simulink model "Synchronousfor2016a"  (R2016a)
settings: Solver=VariableStepAuto  SolverMode=SingleTasking  StartTime=0.0  StopTime=1  MaxStep=1e-4  RelTol=1e-3
undefined symbols (not defined in the file or in its folder): powergui
libraries: powerlib x3, simulink x1
settings Model: Creator=80573  LastModifiedBy=B210b
settings DebuggingCC: SFUnexpectedBacktrackingDiag=error  SFNoUnconditionalDefaultTransitionDiag=error
settings GRTTargetCC: TargetLangStandard=C99 (ISO)  GeneratePreprocessorConditionals=Use local settings
settings ConfigComp: CovMetricSettings=dwe  CovHtmlReporting=off  CovSaveCumulativeToWorkspaceVar=off  CovSaveSingleToWorkspaceVar=off  CovExternalEMLEnable=on

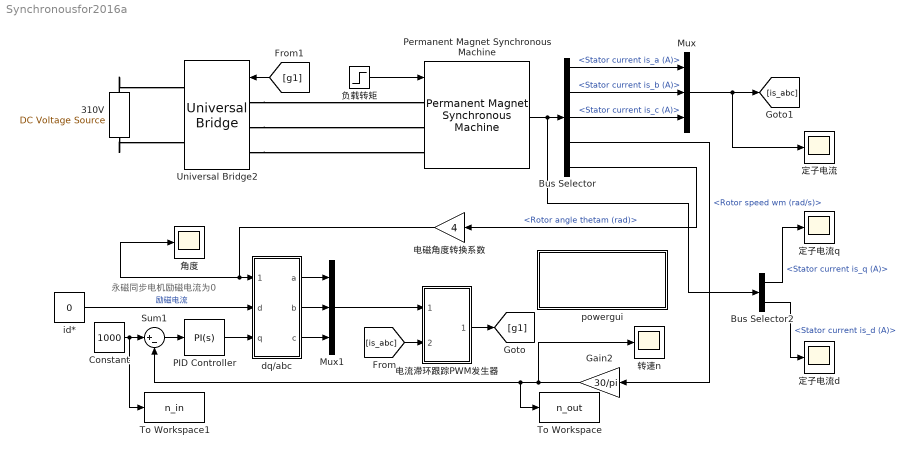
== system Synchronousfor2016a ==
  note: 永磁同步电机励磁电流为0
  310V : powerlib/Electrical Sources/DC Voltage Source  Amplitude=310  Measurements=None
  Bus Selector : BusSelector  OutputSignals=Stator current is_a (A),Stator current is_b (A),Stator current is_c (A),Rotor speed wm (rad/s),Rotor angle thetam (rad)
  Bus Selector2 : BusSelector  OutputSignals=Stator current is_q (A),Stator current is_d (A)
  Constant : Constant  Value=1000
  Gain2 : Gain  Gain=30/pi
  Mux : Mux  Inputs=3
  Mux1 : Mux  Inputs=3
  PID Controller : simulink/Continuous/PID Controller  Controller=PI  Form=Parallel  TimeDomain=Continuous-time  SampleTime=-1  IntegratorMethod=Forward Euler  FilterMethod=Forward Euler  ControllerParametersSource=internal  P=0.05  I=8  D=0  UseFilter=on  N=100  InitialConditionSource=internal  InitialConditionForIntegrator=0  InitialConditionForFilter=0  DifferentiatorICPrevScaledInput=0  ExternalReset=none  TrackingMode=off  Kt=1  LimitOutput=off  UpperSaturationLimit=200  LowerSaturationLimit=-inf  LinearizeAsGain=on  AntiWindupMode=none  Kb=1  POutMin=[]  POutMax=[]  IOutMin=[]  IOutMax=[]  DOutMin=[]  DOutMax=[]  NOutMin=[]  NOutMax=[]  SumOutMin=[]  SumOutMax=[]  SaturationOutMin=[]  SaturationOutMax=[]  PParamMin=[]  PParamMax=[]  IParamMin=[]  IParamMax=[]  DParamMin=[]  DParamMax=[]  NParamMin=[]  NParamMax=[]  KbParamMin=[]  KbParamMax=[]  KtParamMin=[]  KtParamMax=[]  KbOutMin=[]  KbOutMax=[]  KtOutMin=[]  KtOutMax=[]  IntegratorOutMin=[]  IntegratorOutMax=[]  FilterOutMin=[]  FilterOutMax=[]  SumI1OutMin=[]  SumI1OutMax=[]  SumI2OutMin=[]  SumI2OutMax=[]  SumI3OutMin=[]  SumI3OutMax=[]  SumDOutMin=[]  SumDOutMax=[]  DifferentiatorOutMin=[]  DifferentiatorOutMax=[]  IntegratorContinuousStateAttributes=''  IntegratorStateMustResolveToSignalObject=off  IntegratorRTWStateStorageClass=Auto  FilterContinuousStateAttributes=''  FilterStateMustResolveToSignalObject=off  FilterRTWStateStorageClass=Auto
  Permanent Magnet Synchronous Machine : powerlib/Machines/Permanent Magnet Synchronous Machine  NbPhases=3  FluxDistribution=Sinusoidal  RotorType=Salient-pole  MechanicalLoad=Torque Tm  PresetModel=No  ShowDetailedParameters=on  MeasurementBus=off  Resistance=2.785  Inductance=8.5e-3  dqInductances=[0.0085 0.0085]  La=0.02682  MachineConstant=Flux linkage established by magnets (V.s)  Flux=0.175  VoltageCst=126.966  TorqueCst=1.05  Flat=120  Mechanical=[0.001 0.008 4 0]  PolePairs=2  InitialConditions=[0,0, 0,0]  InitialConditions5ph=[0 0 0 0 0 0]  RefAngle=Aligned with phase A axis (original Park)  IterativeDiscreteModel=Trapezoidal non iterative  TsBlock=-1  TsPowergui=0
  Sum1 : Sum  Inputs=|+-
  To Workspace : ToWorkspace  VariableName=n_out  SampleTime=-1
  To Workspace1 : ToWorkspace  VariableName=n_in  SampleTime=-1
  Universal Bridge2 : powerlib/Power Electronics/Universal Bridge  Arms=3  SnubberResistance=1e5  SnubberCapacitance=inf  Device=IGBT / Diodes  Ron=1e-3  Lon=0  ForwardVoltages="[  0  0  ]"  ForwardVoltage=0  GTOparameters=[ 10e-6 , 20e-6 ]  IGBTparameters=[ 1e-6 , 2e-6 ]  Measurements=None  Measurements_2=None  converterType=Rectifier
  dq/abc : Subsystem
  id* : Constant  Value=0
  powergui : Subsystem  AncestorBlock=powerlib/powergui  DialogController=POWERSYS.PowerSysDialog  InitFcn=powergui( 'InitFcn_Callback' , gcb , 0 , [ ] );  mask(PSB option menu block){SimulationMode=Continuous, SampleTime=0.00001, frequency=50, Iterations=50, frequencyindice=0, Pbase=100e6, ErrMax=1e-4, UnitsV=kV, UnitsW=MW, buscounter=0, FunctionMessages=off, echomessages=off, EnableUseOfTLC=off, CurrentSourceSwitches=off, DisableSnubberDevices=off, DisableRonSwitches=off, DisableVfSwitches=off, DisplayEquations=off, AutomaticDiscreteSolvers=off, SolverType=Tustin/Backward Euler (TBE), Interpol=off, ExternalGateDelay=off, methode=off, Ts=100, x0status=zero, SPID=on, SwTol=0, HookPort=off, NonlinearTolerance=1e-4, nMaxIteration=100, ContinueOnMaxIteration=off, RestoreLinks=warning, ResistiveCurrentMeasurement=off, Frange=[0:2:500], Ylog=off, Xlog=on, ShowGrid=off, save=off, variable=ZData, structure=0, ZoomFFT=on, StartTime=0.0, cycles=1, DisplayStyle=1, fundamental=60, FreqAxis=off, MaxFrequency=1000, frequencyindicesteady=1, RmsSteady=1, display=off}
      mask prompts: SimulationMode "Simulation type:"; SampleTime "Sample time (s):"; frequency "Frequency (Hz):"; Iterations "Max iterations"; frequencyindice "Frequency (Hz)"; Pbase "Base power (VA)"; ErrMax "PQ tolerance (pu)"; UnitsV "Voltage units"; UnitsW "Power units"; buscounter "Load flow bus counter"; FunctionMessages "Disable Specialized Power Systems warnings"; echomessages "Display Specialized Power Systems compilation messages"; EnableUseOfTLC "Use TLC file when in Accelerator Simulation Mode and for code generation"; CurrentSourceSwitches "Disable ideal switching"; DisableSnubberDevices "Disable snubbers in switching devices"; DisableRonSwitches "Disable Ron resistances in switching devices"; DisableVfSwitches "Disable forward voltages in switching devices"; DisplayEquations "Display circuit differential equations"; AutomaticDiscreteSolvers "Automatically handle Discrete solver and Advanced tab solver settings of blocks"; SolverType "Discrete solver"; Interpol "Interpolate switching events"; ExternalGateDelay "Use time-stamped gate signals"; methode "Store switching topologies"; Ts "Buffer size (MBytes):"; x0status "Start simulation with initial electrical states from:"; SPID "Use ideal switching devices"; SwTol "Switch tolerance"; HookPort "Allow multiple powergui blocks"; NonlinearTolerance "Solver tolerance"; nMaxIteration "Maximum number of iterations"; ContinueOnMaxIteration "Continue Simulation if maximum number of iterations is reached"; RestoreLinks "Restore disabled links of Simscape Power Systems ST blocks:"; ResistiveCurrentMeasurement "Use non ideal current measurement blocks (1e-4Ohm internal resistance)"; Frange "Frequency Range"; Ylog "Log impedance"; Xlog "log Frequency"; ShowGrid "grid"; save "Save Data To Workspace"; variable "Variable Name"; structure "Structure Name (PSBFFTSCOPE)"; ZoomFFT "ZoomFFT (PSBFFTSCOPE)"; StartTime "Start Time (PSBFFTSCOPE)"; cycles "Cycles (PSBFFTSCOPE)"; DisplayStyle "Display style (PSBFFTSCOPE)"; fundamental "Fundamental (PSBFFTSCOPE)"; FreqAxis "Frequency Axis (PSBFFTSCOPE)"; MaxFrequency "Max Frequency (PSBFFTSCOPE)"; frequencyindicesteady "Frequency indice (STEADYSTATE)"; RmsSteady "RMS display (STEADYSTATE)"; display "Display Results"
      mask help: Set simulation type, simulation parameters, and preferences.
      mask init:
      | dispMessage = powergui('MaskInitialization',gcb,SimulationMode,SampleTime);
      settings: PreSaveFcn=powergui( 'PreSaveFcn_Callback' , gcb , [ ] , [ ] );  OpenFcn=sps_rtmsupport('OpenFcn',gcbh)
      mask Help: helpview(psbhelp)
      mask TypeOptions SimulationMode: Continuous | Discrete | Phasor
      mask Callback SimulationMode: powergui('SimulationType',[],[],gcb);
      mask TypeOptions UnitsV: V | kV
      mask TypeOptions UnitsW: W | kW | MW
      mask Callback CurrentSourceSwitches: powergui('SimulationType',[],[],gcb);
      mask Callback AutomaticDiscreteSolvers: powergui('SimulationType',[],[],gcb);
      mask TypeOptions SolverType: Tustin/Backward Euler (TBE) | Tustin | Backward Euler
      mask Callback SolverType: powergui('SimulationType',[],[],gcb);
      mask Callback Interpol: powergui('SimulationType',[],[],gcb);
      mask Callback ExternalGateDelay: powergui('SimulationType',[],[],gcb);
      mask Callback methode: powergui('SimulationType',[],[],gcb);
      mask TypeOptions x0status: blocks | steady | zero
      mask TypeOptions RestoreLinks: yes | warning | no
      mask Callback display: sps_rtmsupport('parametereditingmodes',gcbh) % Will be executed last in parameter callbacks to ensure mask enable consistency
      mask DialogControl AutoSolverNote Prompt: The Simulation type parameter is governed by Simulink. To access the Powergui solver settings, unselect auto (Automatic solver selection) solver in the Simulink solver options.
      mask DialogControl SteadyState Prompt: Steady-State
      mask DialogControl SteadyState Callback:
      | close_system(gcb)
      | power_steadystate(bdroot(gcb),gcb);
      mask DialogControl InitialState Prompt: Initial State
      mask DialogControl InitialState Callback:
      | close_system(gcb)
      | power_initstates(bdroot(gcb),gcb)
      mask DialogControl MachineInitialization Prompt: Machine Initialization
      mask DialogControl MachineInitialization Callback:
      | close_system(gcb)
      | power_loadflow(bdroot(gcb),gcb)
      mask DialogControl ImpedanceMeasurement Prompt: Impedance Measurement
      mask DialogControl ImpedanceMeasurement Callback:
      | close_system(gcb)
      | power_zmeter(bdroot(gcb),gcb)
      mask DialogControl FFTAnalysis Prompt: FFT Analysis
      mask DialogControl FFTAnalysis Callback:
      | close_system(gcb)
      | power_fftscope(bdroot(gcb),gcb)
      mask DialogControl LinearSystemAnalyzer Prompt: Use Linear System Analyzer
      mask DialogControl LinearSystemAnalyzer Callback:
      | close_system(gcb)
      | power_ltiview(bdroot(gcb),gcb)
      mask DialogControl HysteresisDesign Prompt: Hysteresis Design
      mask DialogControl HysteresisDesign Callback:
      | close_system(gcb)
      | power_hysteresis(bdroot(gcb),gcb)
      mask DialogControl RLCLineParameters Prompt: RLC Line Parameters
      mask DialogControl RLCLineParameters Callback:
      | close_system(gcb)
      | power_lineparam(bdroot(gcb),gcb)
      mask DialogControl GenerateReprot Prompt: Generate Report
      mask DialogControl GenerateReprot Callback:
      | close_system(gcb)
      | power_report(bdroot(gcb),gcb)
      mask DialogControl Control14 Prompt: Customize SPS blocks
      mask DialogControl Control14 Callback:
      | close_system(gcb);
      | power_customize;
      mask DialogControl LoadFlow Prompt: Load Flow
      mask DialogControl LoadFlow Callback:
      | close_system(gcb)
      | power_loadflow('-v2',bdroot(gcb))
      mask DialogControl Container14 Prompt: Load flow settings
      mask DialogControl Solver Prompt: Solver
      mask DialogControl SolverDetails Prompt: Solver details for nonlinear elements
      mask Display: color('blue'),disp(dispMessage)
  定子电流 : Scope
  定子电流d : Scope
  定子电流q : Scope
  电流滞环跟踪PWM发生器 : Subsystem
  电磁角度转换系数 : Gain  Gain=4
  角度 : Scope
  负载转矩 : Step  Time=0.02  Before=4  After=10  SampleTime=0
  转速n : Scope
  wires:
  负载转矩/1 -> Permanent Magnet Synchronous Machine/1
  Permanent Magnet Synchronous Machine/1 -> Bus Selector2/1, Bus Selector/1
  Bus Selector/1 -> Mux/1  "<Stator current is_a (A)>"
  Bus Selector/2 -> Mux/2  "<Stator current is_b (A)>"
  Bus Selector/3 -> Mux/3  "<Stator current is_c (A)>"
  Bus Selector/4 -> Gain2/1  "<Rotor speed wm (rad/s)>"
  Bus Selector/5 -> 电磁角度转换系数/1  "<Rotor angle thetam (rad)>"
  Constant/1 -> To Workspace1/1, Sum1/1
  id*/1 -> dq/abc/2(d)  "励磁电流"
  Mux/1 -> 定子电流/1, [is_abc]
  电流滞环跟踪PWM发生器/1(pulse) -> [g1]
  dq/abc/1(a) -> Mux1/1
  dq/abc/2(b) -> Mux1/2
  dq/abc/3(c) -> Mux1/3
  Mux1/1 -> 电流滞环跟踪PWM发生器/1(Iabc*)
  [is_abc] -> 电流滞环跟踪PWM发生器/2(Iabc)
  电磁角度转换系数/1 -> 角度/1, dq/abc/1(theta)
  [g1] -> Universal Bridge2/1
  Sum1/1 -> PID Controller/1
  PID Controller/1 -> dq/abc/3(q)
  Bus Selector2/1 -> 定子电流q/1  "<Stator current is_q (A)>"
  Bus Selector2/2 -> 定子电流d/1  "<Stator current is_d (A)>"
  Gain2/1 -> To Workspace/1, Sum1/2, 转速n/1
  connections:
  310V/LConn1 -- Universal Bridge2/RConn2
  Universal Bridge2/LConn1 -- Permanent Magnet Synchronous Machine/LConn1
  310V/RConn1 -- Universal Bridge2/RConn1
  Universal Bridge2/LConn3 -- Permanent Magnet Synchronous Machine/LConn3
  Universal Bridge2/LConn2 -- Permanent Magnet Synchronous Machine/LConn2

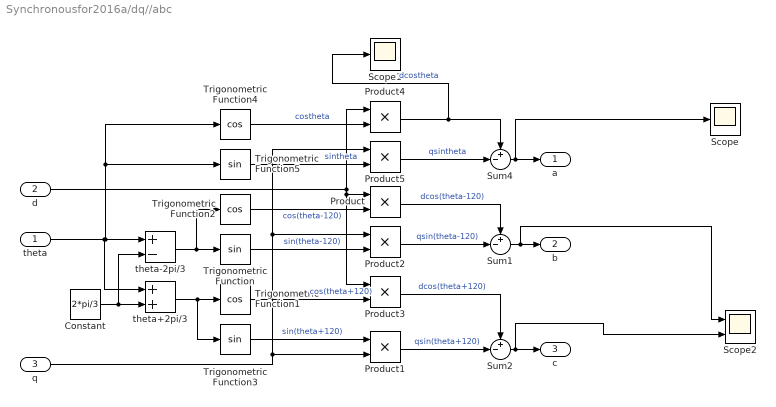
== system Synchronousfor2016a/dq//abc ==
  theta : Inport
  d : Inport  Port=2
  q : Inport  Port=3
  Constant : Constant  Value=2*pi/3
  Product{,1..5} (6 alike) : Product
  Scope : Scope
  Scope1 : Scope
  Scope2 : Scope  NumInputPorts=2
  Sum1 : Sum  Inputs=+-|
  Sum2 : Sum  Inputs=+-|
  Sum4 : Sum  Inputs=+-|
  Trigonometric Function : Trigonometry
  Trigonometric Function1 : Trigonometry  Operator=cos
  Trigonometric Function2 : Trigonometry  Operator=cos
  Trigonometric Function3 : Trigonometry
  Trigonometric Function4 : Trigonometry  Operator=cos
  Trigonometric Function5 : Trigonometry
  theta+2pi/3 : Sum
  theta-2pi/3 : Sum  Inputs=+-
  a : Outport
  b : Outport  Port=2
  c : Outport  Port=3
  wires:
  Trigonometric Function5/1 -> Product5/2  "sintheta"
  Product/1 -> Sum1/1  "dcos(theta-120)"
  Trigonometric Function1/1 -> Product3/2  "cos(theta+120)"
  Product3/1 -> Sum2/1  "dcos(theta+120)"
  d/1 -> Product/1, Product3/1, Product4/1
  Constant/1 -> theta+2pi/3/2, theta-2pi/3/2
  theta/1 -> Trigonometric Function4/1, Trigonometric Function5/1, theta-2pi/3/1, theta+2pi/3/1
  theta+2pi/3/1 -> Trigonometric Function3/1, Trigonometric Function1/1
  q/1 -> Product5/1, Product2/1, Product1/2
  Trigonometric Function/1 -> Product2/2  "sin(theta-120)"
  Product4/1 -> Scope1/1, Sum4/1  "dcostheta"
  Product5/1 -> Sum4/2  "qsintheta"
  theta-2pi/3/1 -> Trigonometric Function2/1, Trigonometric Function/1
  Product1/1 -> Sum2/2  "qsin(theta+120)"
  Trigonometric Function2/1 -> Product/2  "cos(theta-120)"
  Sum4/1 -> Scope/1, a/1
  Sum1/1 -> Scope2/1, b/1
  Trigonometric Function4/1 -> Product4/2  "costheta"
  Trigonometric Function3/1 -> Product1/1  "sin(theta+120)"
  Product2/1 -> Sum1/2  "qsin(theta-120)"
  Sum2/1 -> Scope2/2, c/1

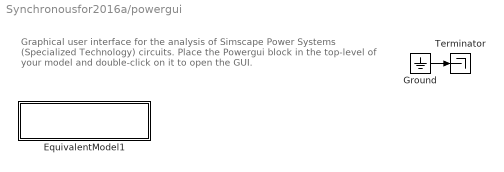
== system Synchronousfor2016a/powergui ==
  note: Graphical user interface for the analysis of
      | Simscape Power Systems (Specialized Technology) circuits.
      | Place the Powergui block in the top-level of your model and double-click
      | on it to open the GUI.
  EquivalentModel1 : Subsystem  mask{SwTol=0}
      mask prompts: SwTol "SwitchTolerance"
      mask init:
      | S  = GetDataForEquivalentModel('SPID',gcbh,SwTol);
      mask Display:
      | color('blue')
      | disp('EQUIVALENT CIRCUIT\nSPID')
  Ground : Ground
  Terminator : Terminator
  wires:
  Ground/1 -> Terminator/1

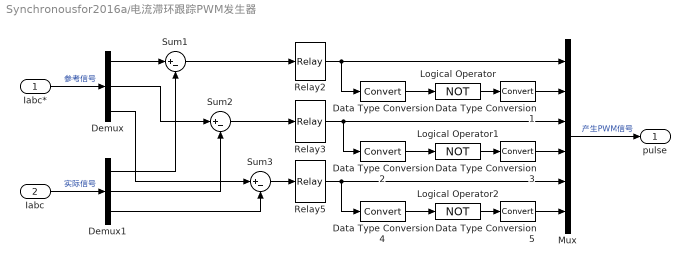
== system Synchronousfor2016a/电流滞环跟踪PWM发生器 ==
  Iabc* : Inport
  Iabc : Inport  Port=2
  Data Type Conversion{,1..5} (6 alike) : DataTypeConversion
  Demux : Demux  Outputs=3
  Demux1 : Demux  Outputs=3
  Logical Operator : Logic  Operator=NOT  Inputs=1  AllPortsSameDT=off
  Logical Operator1 : Logic  Operator=NOT  Inputs=1  AllPortsSameDT=off
  Logical Operator2 : Logic  Operator=NOT  Inputs=1  AllPortsSameDT=off
  Mux : Mux  Inputs=6
  Relay2 : Relay  OnSwitchValue=0.1  OffSwitchValue=-0.1  ZeroCross=off
  Relay3 : Relay  OnSwitchValue=0.1  OffSwitchValue=-0.1  ZeroCross=off
  Relay5 : Relay  OnSwitchValue=0.1  OffSwitchValue=-0.1  ZeroCross=off
  Sum1 : Sum  Inputs=|+-
  Sum2 : Sum  Inputs=|+-
  Sum3 : Sum  Inputs=|+-
  pulse : Outport
  wires:
  Relay2/1 -> Data Type Conversion/1, Mux/1
  Data Type Conversion/1 -> Logical Operator/1
  Logical Operator/1 -> Data Type Conversion1/1
  Data Type Conversion1/1 -> Mux/2
  Mux/1 -> pulse/1  "产生PWM信号"
  Sum1/1 -> Relay2/1
  Demux/1 -> Sum1/1
  Demux1/3 -> Sum3/2
  Iabc/1 -> Demux1/1  "实际信号"
  Iabc*/1 -> Demux/1  "参考信号"
  Sum2/1 -> Relay3/1
  Logical Operator1/1 -> Data Type Conversion3/1
  Data Type Conversion3/1 -> Mux/4
  Data Type Conversion2/1 -> Logical Operator1/1
  Relay3/1 -> Data Type Conversion2/1, Mux/3
  Logical Operator2/1 -> Data Type Conversion5/1
  Data Type Conversion5/1 -> Mux/6
  Data Type Conversion4/1 -> Logical Operator2/1
  Relay5/1 -> Data Type Conversion4/1, Mux/5
  Sum3/1 -> Relay5/1
  Demux/2 -> Sum2/1
  Demux1/1 -> Sum1/2
  Demux1/2 -> Sum2/2
  Demux/3 -> Sum3/1

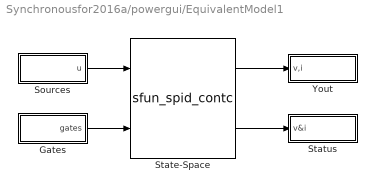
== system Synchronousfor2016a/powergui/EquivalentModel1 ==
  Gates : Subsystem
  Sources : Subsystem
  State-Space : S-Function  FunctionName=sfun_spid_contc  Parameters=S.Mg, [S.nb.x S.nb.u S.nb.y S.nb.s], S.x0, S.MgColNames, S.SwitchVf, S.SwitchType, S.SwitchGateInitialValue, S.SwitchTolerance,S.SaveMatrices,S.BufferSize  SFunctionDeploymentMode=off  EnableBusSupport=off
  Status : Subsystem
  Yout : Subsystem
  wires:
  State-Space/1 -> Yout/1(v,i)
  State-Space/2 -> Status/1(v&i)
  Sources/1(u) -> State-Space/1
  Gates/1(gates) -> State-Space/2

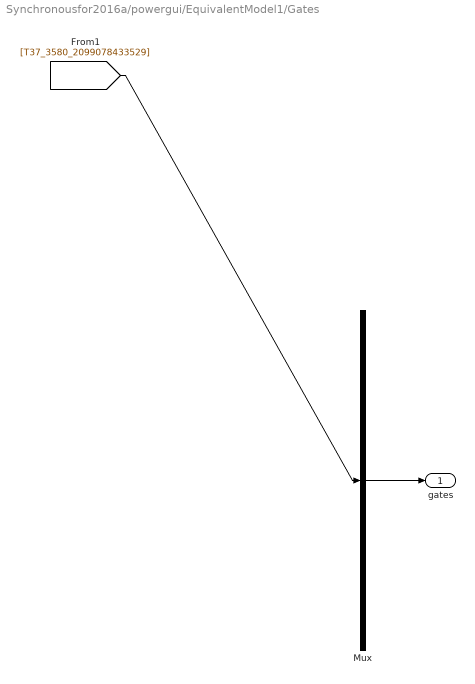
== system Synchronousfor2016a/powergui/EquivalentModel1/Gates ==
  Mux : Mux  Inputs=1
  gates : Outport
  wires:
  Mux/1 -> gates/1
  [T37_3580_2099078433529] -> Mux/1

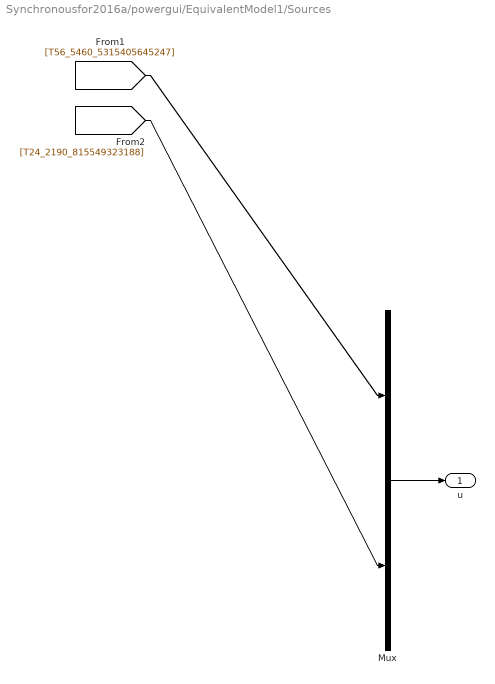
== system Synchronousfor2016a/powergui/EquivalentModel1/Sources ==
  Mux : Mux  Inputs=[2 1]
  u : Outport
  wires:
  Mux/1 -> u/1
  [T56_5460_5315405645247] -> Mux/1
  [T24_2190_815549323188] -> Mux/2

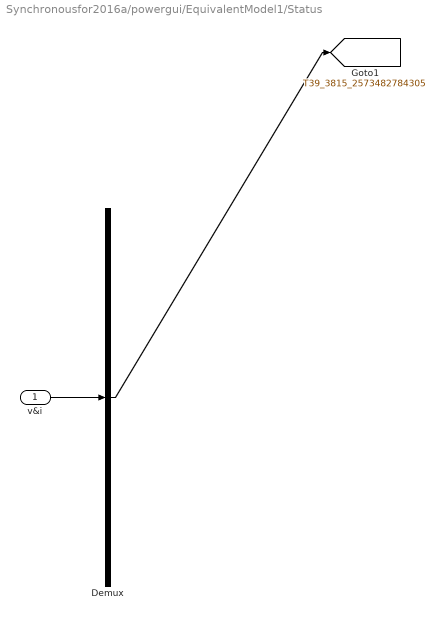
== system Synchronousfor2016a/powergui/EquivalentModel1/Status ==
  v&i : Inport
  Demux : Demux  Outputs=1
  tag scope: T39_3815_2573482784305=global
  wires:
  v&i/1 -> Demux/1
  Demux/1 -> [T39_3815_2573482784305]

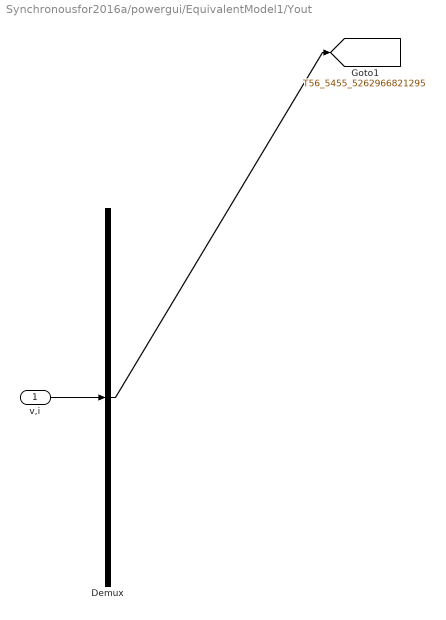
== system Synchronousfor2016a/powergui/EquivalentModel1/Yout ==
  v,i : Inport
  Demux : Demux  Outputs=1
  tag scope: T56_5455_5262966821295=global
  wires:
  v,i/1 -> Demux/1
  Demux/1 -> [T56_5455_5262966821295]
